simulink model "mpc555_v12_sade_ve_duzenli"  (Simulink 7.0)
settings: Solver=FixedStepDiscrete  StartTime=0.0  StopTime=inf  FixedStep=dt_sys  RelTol=1e-3
PreLoadFcn:
  | RTWConfigurationCB('preloadfcn', bdroot);
InitFcn:
  | % START RTW CONFIGURATION CODE %
  | RTWConfigurationCB('rtw_target_initfcn',gcs);
  | % END RTW CONFIGURATION CODE %
values from neighbouring files (symbols this model uses):
  dt = 1/50    (= 0.02)    [init_par.m]
  dt_serial_RX1 = dt/120    (= 0.000166666666667)    [init_par.m]
  dt_serial_TX2 = dt/120    (= 0.000166666666667)    [init_par.m]
undefined symbols (not defined in the file or in its folder): DiscIntNeverNeededParam
libraries: aerolibconvert2 x9, mpc555drivers x5, simulink x1
(part 2 of 2)

== matlab function Stystem Counter ==
  data: count output inherited
function count  = fcn
% This block supports the Embedded MATLAB subset.
% See the help menu for details. 
persistent counter

if isempty(counter)
    counter =uint16(0);
end

if(counter==65535)
    counter=uint16(0);
end
counter=counter+1;
count=counter;

== matlab function Embedded MATLAB Function ==
  data: a input inherited; P1 output inherited; P2 output inherited; P3 output inherited; b input inherited; c input inherited
function [P1,P2,P3] = fcn(a, b, c)
% This block supports the Embedded MATLAB subset.
% See the help menu for details. 
P1temp = zeros(4,1);
P2temp = zeros(4,1);
P3temp = zeros(4,1);
xP1 = zeros(4,1);
xP2 = zeros(4,1);
xP3 = zeros(4,1);
P1temp(1:4) = typecast(double(a),'int16');
P2temp(1:4) = typecast(double(b),'int16');
P3temp(1:4) = typecast(double(c),'int16');

xP1(1)=P1temp(4);
xP1(2)=P1temp(3);
xP1(3)=P1temp(2);
xP1(4)=P1temp(1);
xP2(1)=P2temp(4);
xP2(2)=P2temp(3);
xP2(3)=P2temp(2);
xP2(4)=P2temp(1);
xP3(1)=P3temp(4);
xP3(2)=P3temp(3);
xP3(3)=P3temp(2);
xP3(4)=P3temp(1);

P1=xP1;
P2=xP2;
P3=xP3;

== matlab function Receive_IMU_Data/Receive Buffer1 ==
  data: Data input uint8; bytes output uint8; endinx output double; Num input double; inbuflen output double
function [bytes, endinx, inbuflen] = buffer(Data, Num)
%inbuflenSC1 length parameter for input buffer
inbuflenSC1 = 170;

persistent rdata inx

% Initialize persistent data
if isempty(rdata)
    rdata = uint8(zeros(inbuflenSC1,1));
end
if isempty(inx)
    inx = 1;
end

% If Data exists
if (Num > 0)
    for inxdata = 1:Num        
        % Grap Data bytes    
        rdata(inx) = Data(inxdata);
        inx = inx + 1;
        if (inx > inbuflenSC1)
            inx = 1;
        end
    end %for
end %if

endinx = inx;
bytes = rdata;
inbuflen = inbuflenSC1;

== matlab function Receive_IMU_Data/IMU B2D ==
  data: dvalid input double; accX output uint16; accY output uint16; accZ output uint16; gyroX output uint16; gyroY output uint16; gyroZ output uint16; magX output uint16; magY output uint16; magZ output uint16; temp output uint16; alt output uint16; airs output uint16; bytes input uint8; temp1 output inherited; temp2 output inherited; temp3 output inherited; temp4 output inherited; temp5 output inherited; temp6 output inherited; temp7 output inherited; temp8 output inherited
function [ accX,accY,accZ,gyroX,gyroY,gyroZ,magX,magY,magZ,temp,alt,airs, temp1, temp2, temp3,temp4, temp5, temp6,temp7, temp8 ] = B2D(dvalid,bytes)

persistent XaccX XaccY XaccZ XgyroX XgyroY XgyroZ XmagX XmagY XmagZ Xtemp Xalt Xairs Xtemp1 Xtemp2 Xtemp3 Xtemp4 Xtemp5 Xtemp6 Xtemp7 Xtemp8 
% Initialize persistent data
if isempty(XaccX)
   XaccX=uint16(0);
end
if isempty(XaccY)
   XaccY=uint16(0);
end
if isempty(XaccZ)
   XaccZ=uint16(0);
end
if isempty(XgyroX)
   XgyroX=uint16(0);
end
if isempty(XgyroY)
   XgyroY=uint16(0);
end
if isempty(XgyroZ)
   XgyroZ=uint16(0);
end
if isempty(XmagX)
   XmagX=uint16(0);
end
if isempty(XmagY)
   XmagY=uint16(0);
end
if isempty(XmagZ)
   XmagZ=uint16(0);
end
if isempty(Xtemp)
   Xtemp=uint16(0);
end
if isempty(Xalt)
   Xalt=uint16(0);
end
if isempty(Xairs)
   Xairs=uint16(0);
end
if isempty(Xtemp1)
   Xtemp1=uint16(0);
end
if isempty(Xtemp2)
   Xtemp2=uint16(0);
end
if isempty(Xtemp3)
   Xtemp3=uint16(0);
end
if isempty(Xtemp4)
   Xtemp4=uint16(0);
end
if isempty(Xtemp5)
   Xtemp5=uint16(0);
end
if isempty(Xtemp6)
   Xtemp6=uint16(0);
end
if isempty(Xtemp7)
   Xtemp7=uint16(0);
end
if isempty(Xtemp8)
   Xtemp8=uint16(0);
end
% accX = zeros(1,1,'uint16');
% accY = zeros(1,1,'uint16');
% accZ = zeros(1,1,'uint16');
% gyroX = zeros(1,1,'uint16');
% gyroY =zeros(1,1,'uint16');
% gyroZ = zeros(1,1,'uint16');
% magX = zeros(1,1,'uint16');
% magY = zeros(1,1,'uint16');
% magZ = zeros(1,1,'uint16');
% temp = zeros(1,1,'uint16');
% alt = zeros(1,1,'uint16');
% airs = zeros(1,1,'uint16');

if (dvalid == 1)
    
  %accX(1)=double(typecast(bytes(2:-1:1),'uint16'));
  
  %accX=[bytes(2); bytes(1)];
    YaccX= typecast(bytes(2:-1:1),'uint16');
    YaccY= typecast(bytes(4:-1:3),'uint16');
    YaccZ= typecast(bytes(6:-1:5),'uint16');
    YgyroX= typecast(bytes(8:-1:7),'uint16');
    YgyroY= typecast(bytes(10:-1:9),'uint16');
    YgyroZ= typecast(bytes(12:-1:11),'uint16');
    YmagX= typecast(bytes(14:-1:13),'uint16');
    YmagY= typecast(bytes(16:-1:15),'uint16');
    YmagZ= typecast(bytes(18:-1:17),'uint16');
    Ytemp= typecast(bytes(20:-1:19),'uint16');
    Yalt= typecast(bytes(22:-1:21),'uint16');
    Yairs= typecast(bytes(24:-1:23),'uint16');
    Ytemp1= typecast(bytes(26:-1:25),'uint16');
    Ytemp2= typecast(bytes(28:-1:27),'uint16');
    Ytemp3= typecast(bytes(30:-1:29),'uint16');
    Ytemp4= typecast(bytes(32:-1:31),'uint16');
    Ytemp5= typecast(bytes(34:-1:33),'uint16');
    Ytemp6= typecast(bytes(36:-1:35),'uint16');
    Ytemp7= typecast(bytes(38:-1:37),'uint16');
    Ytemp8= typecast(bytes(40:-1:39),'uint16');
    
    XaccX=YaccX(1) ;
    XaccY=YaccY(1) ;
    XaccZ=YaccZ(1) ;
    XgyroX=YgyroX(1);
    XgyroY=YgyroY(1);
    XgyroZ=YgyroZ(1);
    XmagX=YmagX(1);
    XmagY=YmagY(1);
    XmagZ=YmagZ(1); 
    Xtemp=Ytemp(1);
    Xalt=Yalt(1);
    Xairs=Yairs(1);
    Xtemp1=Ytemp1(1);
    Xtemp2=Ytemp2(1);
    Xtemp3=Ytemp3(1);
    Xtemp4=Ytemp4(1);
    Xtemp5=Ytemp5(1);
    Xtemp6=Ytemp6(1);
    Xtemp7=Ytemp7(1);
    Xtemp8=Ytemp8(1);
    
    
end
    
    %ivalue = typecast(bytes(24:-1:23),'uint16');
   accX=XaccX ;
   accY=XaccY ;
   accZ=XaccZ ;
   gyroX=XgyroX;
   gyroY=XgyroY;
   gyroZ=XgyroZ;
   magX=XmagX;
   magY=XmagY;
   magZ=XmagZ; 
   temp=Xtemp;
   alt=Xalt;
   airs=Xairs;
   temp1=Xtemp1;
   temp2=Xtemp2;
   temp3=Xtemp3;
   temp4=Xtemp4;
   temp5=Xtemp5;
   temp6=Xtemp6;
    temp7=Xtemp7;
   temp8=Xtemp8;
   % value = uint8(ivalue(1));
%end

== matlab function Receive_IMU_Data/GPS B2D ==
  data: dvalid input inherited; bytes input inherited; Lat_Degrees output inherited; Lat_Mins output uint16; Lat_Fractions output uint16; Lat_Dir output uint16; Lon_Degrees output uint16; Lon_Mins output uint16; Lon_Fractions output uint16; Lon_Dir output uint16; gps_alt output inherited; gps_alt_fraction output inherited; gps_speed output uint16; gps_speed_fraction output uint16; gps_trackangle output uint16; gps_trackangle_fraction output uint16; gps_date output inherited; gps_month output inherited; gps_year output inherited; gps_time_h output double; gps_time_m output inherited; gps_time_s output inherited
function [Lat_Degrees,Lat_Mins,Lat_Fractions,Lat_Dir,Lon_Degrees,Lon_Mins,Lon_Fractions,Lon_Dir,gps_alt, gps_alt_fraction, gps_speed,gps_speed_fraction,gps_trackangle,gps_trackangle_fraction, gps_date, gps_month, gps_year, gps_time_h, gps_time_m, gps_time_s] = B2D(dvalid,bytes)

persistent XLat_Degrees XLat_Mins XLat_Fractions XLat_Dir XLon_Degrees XLon_Mins XLon_Fractions XLon_Dir Xgps_speed Xgps_speed_fraction Xgps_trackangle Xgps_trackangle_fraction Xgps_date Xgps_month Xgps_year Xgps_time_h Xgps_time_m Xgps_time_s Xgps_alt Xgps_alt_fraction

	
% Initialize persistent data
if isempty(XLat_Degrees)
   XLat_Degrees=uint16(0);
end
if isempty(XLat_Mins)
   XLat_Mins=uint16(0);
end
if isempty(XLat_Fractions)
   XLat_Fractions=uint16(0);
end
if isempty(XLat_Dir)
   XLat_Dir=uint16(0);
end
if isempty(XLon_Degrees)
   XLon_Degrees=uint16(0);
end
if isempty(XLon_Mins)
   XLon_Mins=uint16(0);
end
if isempty(XLon_Fractions)
   XLon_Fractions=uint16(0);
end
if isempty(XLon_Dir)
   XLon_Dir=uint16(0);
end
if isempty(Xgps_speed)
   Xgps_speed=uint16(0);
end
if isempty(Xgps_speed_fraction)
   Xgps_speed_fraction=uint16(0);
end
if isempty(Xgps_trackangle)
   Xgps_trackangle=uint16(0);
end
if isempty(Xgps_trackangle_fraction)
   Xgps_trackangle_fraction=uint16(0);
end
if isempty(Xgps_date)
   Xgps_date=uint16(0);
end
if isempty(Xgps_month)
   Xgps_month=uint16(0);
end
if isempty(Xgps_year)
   Xgps_year=uint16(0);
end
if isempty(Xgps_time_h)
   Xgps_time_h=uint16(0);
end
if isempty(Xgps_time_m)
   Xgps_time_m=uint16(0);
end
if isempty(Xgps_time_s)
   Xgps_time_s=uint16(0);
end
if isempty(Xgps_alt)
   Xgps_alt=uint16(0);
end
if isempty(Xgps_alt_fraction)
   Xgps_alt_fraction=uint16(0);
end


% Lat_Degrees = zeros(1,1,'uint16');
% Lat_Mins = zeros(1,1,'uint16');
% Lat_Fractions = zeros(1,1,'uint16');
% Lat_Dir = zeros(1,1,'uint16');
% Lon_Degrees =zeros(1,1,'uint16');
% Lon_Mins = zeros(1,1,'uint16');
% Lon_Fractions = zeros(1,1,'uint16');
% Lon_Dir = zeros(1,1,'uint16');
% gps_speed = zeros(1,1,'uint16');
% gps_speed_fraction = zeros(1,1,'uint16');
% gps_trackangle = zeros(1,1,'uint16');
% gps_trackangle_fraction = zeros(1,1,'uint16');

if (dvalid == 1)
    
  %Lat_Degrees(1)=double(typecast(bytes(2:-1:1),'uint16'));
  
  %Lat_Degrees=[bytes(2); bytes(1)];
    YLat_Degrees= typecast(bytes(2:-1:1),'uint16');
    YLat_Mins= typecast(bytes(4:-1:3),'uint16');
    YLat_Fractions= typecast(bytes(6:-1:5),'uint16');
    YLat_Dir= typecast(bytes(8:-1:7),'uint16');
    YLon_Degrees= typecast(bytes(10:-1:9),'uint16');
    YLon_Mins= typecast(bytes(12:-1:11),'uint16');
    YLon_Fractions= typecast(bytes(14:-1:13),'uint16');
    YLon_Dir= typecast(bytes(16:-1:15),'uint16');
    Ygps_alt= typecast(bytes(18:-1:17),'uint16');
    Ygps_alt_fraction= typecast(bytes(20:-1:19),'uint16');
    Ygps_speed= typecast(bytes(22:-1:21),'uint16');
    Ygps_speed_fraction= typecast(bytes(24:-1:23),'uint16');
    Ygps_trackangle= typecast(bytes(26:-1:25),'uint16');
    Ygps_trackangle_fraction= typecast(bytes(28:-1:27),'uint16');
    Ygps_date= typecast(bytes(30:-1:29),'uint16');
    Ygps_month= typecast(bytes(32:-1:31),'uint16');
    Ygps_year= typecast(bytes(34:-1:33),'uint16');
    Ygps_time_h= typecast(bytes(36:-1:35),'uint16');
    Ygps_time_m= typecast(bytes(38:-1:37),'uint16');
    Ygps_time_s= typecast(bytes(40:-1:39),'uint16');
    
    
    
    XLat_Degrees=YLat_Degrees(1) ;
    XLat_Mins=YLat_Mins(1) ;
    XLat_Fractions=YLat_Fractions(1) ;
    XLat_Dir=YLat_Dir(1);
    XLon_Degrees=YLon_Degrees(1);
    XLon_Mins=YLon_Mins(1);
    XLon_Fractions=YLon_Fractions(1);
    XLon_Dir=YLon_Dir(1);
    Xgps_speed=Ygps_speed(1); 
    Xgps_speed_fraction=Ygps_speed_fraction(1);
    Xgps_trackangle=Ygps_trackangle(1);
    Xgps_trackangle_fraction=Ygps_trackangle_fraction(1);
    Xgps_date=Ygps_date(1);
    Xgps_month=Ygps_month(1);
    Xgps_year=Ygps_year(1);
    Xgps_time_h=Ygps_time_h(1);
    Xgps_time_m=Ygps_time_m(1);
    Xgps_time_s=Ygps_time_s(1);
    Xgps_alt=Ygps_alt(1);
    Xgps_alt_fraction=Ygps_alt_fraction(1);
    
    
end
    
    %ivalue = typecast(bytes(24:-1:23),'uint16');
   Lat_Degrees=XLat_Degrees ;
   Lat_Mins=XLat_Mins ;
   Lat_Fractions=XLat_Fractions ;
   Lat_Dir=XLat_Dir;
   Lon_Degrees=XLon_Degrees;
   Lon_Mins=XLon_Mins;
   Lon_Fractions=XLon_Fractions;
   Lon_Dir=XLon_Dir;
   gps_speed=Xgps_speed; 
   gps_speed_fraction=Xgps_speed_fraction;
   gps_trackangle=Xgps_trackangle;
   gps_trackangle_fraction=Xgps_trackangle_fraction;
   gps_date=Xgps_date;
   gps_month=Xgps_month;
   gps_year=Xgps_year;
   gps_time_h=Xgps_time_h;
   gps_time_m=Xgps_time_m;
   gps_time_s=Xgps_time_s;
   gps_alt=Xgps_alt;
   gps_alt_fraction=Xgps_alt_fraction;
   % value = uint8(ivalue(1));
%end

== matlab function Receive_IMU_Data/Read Buffer2 ==
  data: dvalid output double; imu_data output double; bytes input uint8; endinx input double; inbuflenSC2 input double
function [dvalid, imu_data] = fcn(bytes, endinx, inbuflenSC2)
%inbuflenSC2 length parameter for input buffer

persistent indata inx curinx 


%Constants 
headerlen = 2;
dlen = 40;
cslen = 2;

% Initialize persistent data
if isempty(indata)
    indata = zeros(dlen,1,'uint8');
end
if isempty(inx)
    inx = 1;
end
if isempty(curinx)
    curinx = 1;
end

outbuf = uint8(zeros(dlen,1));

dvalid = uint8(0);
%
while ((endinx ~= 0) && (inx ~= endinx))
    if (curinx == 1)
        if (bytes(inx) == 255) %0xFF
            curinx = curinx + 1;
        else
            curinx=1;
        end       
    elseif (curinx == 2)
        if (bytes(inx) == 251) %0xFB
            curinx = curinx + 1;
        elseif (bytes(inx) == 255) %0xFF
            curinx = 2;
        else
            curinx = 1;
        end
    elseif (curinx == 43)
        if (bytes(inx) == 13) %0x0D
            curinx = curinx + 1;
        else
            curinx = 1;
        end
    elseif (curinx == 44)   % Last data received       
        if (bytes(inx) == 10) %0x0A
            outbuf = indata;    % Copy received data to output buffer            
        %    dvalid = dvalid + uint8(1);         % This data is valid and fresh
            dvalid =uint8(1);         % This data is valid and fresh
        end              
        curinx = 1; % Reset counter             
    else    % Grap Data bytes  
        indata(curinx-headerlen) = bytes(inx);
        curinx = curinx + 1;
    end       
    
    inx = inx + 1;
    if (inx > inbuflenSC2)
        inx = 1;
    end
end

imu_data = outbuf(1:dlen);

== matlab function Butunlesik Seyir Sistemi/Hesaplamalar/INS/GPS Hiz Bilesenleri ==
  data: gpsspeed input double; Vx output double; gpsheading input double; Vy output double
function [Vx,Vy] = fcn(gpsspeed,gpsheading)
%#eml

 Vx=gpsspeed*cos(gpsheading*(3.14159/180.00));
  Vy=gpsspeed*sin(gpsheading*(3.14159/180.00));

== matlab function Butunlesik Seyir Sistemi/Hesaplamalar/INS/Govde-Seyrusefer Eksen Donusumu ==
  data: accx input double; accy input double; accz input double; roll input double; aN output double; pitch input double; yaw input double; aE output double; aD output double
function [aN,aE,aD] = fcn(accx,accy,accz,roll,pitch,yaw)
%#eml

persistent Macc  sample_counter ax ay az aN_correction aE_correction aD_correction cal_finished Y;

num_of_sample=100;

% Initialize persistent data
if isempty(Macc)
    Macc = [0;0;0];
end

if isempty(sample_counter)
    sample_counter = 0;
end

if isempty(ax)
    ax = 0;
end

if isempty(ay)
    ay = 0;
end

if isempty(az)
    az = 0;
end

if isempty(aN_correction)
    aN_correction = 0;
end
if isempty(aE_correction)
    aE_correction = 0;
end
if isempty(aD_correction)
    aD_correction = 0;
end
if isempty(cal_finished)
    cal_finished = 0;
end
if isempty(Y)
    Y =[0;0;0];
end

if(sample_counter<num_of_sample)
   if(sample_counter>10)
   ax=ax+accx;
   ay=ay+accy;
   az=az+accz;
   end
   sample_counter=sample_counter+1;
end

%%%%%%%%%%%%%%%%%%%Calibration Routine%%%%%%%%%%%%%%%%%%%%%%
if(sample_counter==num_of_sample)
    aN_correction=ax/(num_of_sample-11);
    aE_correction=ay/(num_of_sample-11);
    aD_correction=az/(num_of_sample-11);
    cal_finished=1;
    sample_counter=sample_counter+1;
end
%%%%%%%%%%%%%%%%%%%%%%%%%%%%%%%%%%%%%%%%%%%%%%%%%%%%%%%%%%%%%

if(cal_finished==1)
Macc(1,1)=accx;
Macc(2,1)=-accy;
Macc(3,1)=accz;

%DCM matris Body to Navigation Frame
M2=[ cos(pitch)*cos(yaw)   (sin(roll)*sin(pitch)*cos(yaw)- cos(roll)*sin(yaw))    (cos(roll)*sin(pitch)*cos(yaw)+ sin(roll)*sin(yaw)) ;
    cos(pitch)*sin(yaw)    (sin(roll)*sin(pitch)*sin(yaw)+ cos(roll)*cos(yaw))    (cos(roll)*sin(pitch)*sin(yaw)- sin(roll)*cos(yaw));
    -sin(pitch)                         (sin(roll)*cos(pitch))                                (cos(roll)*cos(pitch))];

% M2=[ 1   tan(pitch)*sin(roll)    tan(pitch)*cos(roll)  ;
%     0       cos(roll)                -sin(roll)       ;
%     0   (sin(roll)/cos(pitch))  (cos(roll)/cos(pitch))];

Y=M2*Macc;
end
aN=Y(1,1)-aN_correction;
aE=Y(2,1)-aE_correction;
aD=-((Y(3,1))-aD_correction);

== matlab function Butunlesik Seyir Sistemi/Gercek Birimleri Hesapla/Manyetometre ==
  data: RAWmagX input double; magX output double; RAWmagY input double; RAWmagZ input double; magY output double; magZ output double; X_MIN output double; X_MAX output double; Y_MIN output double; Y_MAX output double; Z_MIN output double; Z_MAX output double; XScale output double; YScale output double; Xoff output double; Yoff output double; CAL_EN input double

function [magX,magY,magZ,X_MIN, X_MAX, Y_MIN, Y_MAX, Z_MIN, Z_MAX, XScale,YScale, Xoff,Yoff ] = fcn(RAWmagX,RAWmagY,RAWmagZ, CAL_EN )
%#eml


persistent RmagX_MIN RmagX_MAX RmagY_MIN RmagY_MAX RmagZ_MIN RmagZ_MAX XRange YRange ZRange Xsf Ysf Zsf X_off Y_off Z_off Xold Yold Zold RAWmX RAWmY RAWmZ first_time cal_done count
%persistent Xtemp Ytemp Ztemp
%persistent roll pitch

% Initialize persistent data
if isempty(RmagX_MIN)
    RmagX_MIN = double(4095);
end

if isempty(RmagX_MAX)
    RmagX_MAX = double(0);
end

if isempty(RmagY_MIN)
    RmagY_MIN = double(4095);
end

if isempty(RmagY_MAX)
    RmagY_MAX =double(0);
end

if isempty(RmagZ_MIN)
    RmagZ_MIN = double(4095);
end

if isempty(RmagZ_MAX)
    RmagZ_MAX = double(0);
end

if isempty(Xsf)
    Xsf = double(1);
end
if isempty(Ysf)
    Ysf = double(1);
end
if isempty(Zsf)
    Zsf = double(1);
end
if isempty(X_off)
    X_off = double(136);
end
if isempty(Y_off)
    Y_off = double(136);
end
if isempty(Z_off)
    Z_off = double(136);
end

if isempty(Xold)
    Xold = RAWmagX;
end
if isempty(Yold)
    Yold = RAWmagY;
end
if isempty(Zold)
    Zold = RAWmagZ;
end

if isempty(RAWmX)
    RAWmX = RAWmagX;
end

if isempty(RAWmY)
    RAWmY = RAWmagY;
end

if isempty(RAWmZ)
    RAWmZ = RAWmagZ;
end

if isempty(XRange)
    XRange =double(192);
end

if isempty(YRange)
    YRange =double(160);
end

if isempty(ZRange)
    ZRange =double(192);
end

if isempty(first_time)
    first_time = double(1);
end

if isempty(cal_done)
    cal_done = double(0);
end

if isempty(count)
    count = uint16(0);
end
%%%%%%%%%%%%%%Filter the data%%%%%%%%%%%%%%%%
if(count<100)
    count=count+1;
end
    
   if(count>=100)
       if(abs(RAWmagX-Xold)< 50)
            RAWmX=RAWmagX;
            Xold=RAWmX;
        else
            RAWmX=Xold;
        end

        if(abs(RAWmagY-Yold)< 50)
            RAWmY=RAWmagY;
            Yold=RAWmY;
        else
            RAWmY=Yold;
        end

        if(abs(RAWmagZ-Zold)< 50)
            RAWmZ=RAWmagZ;
            Zold=RAWmZ;
        else
            RAWmZ=Zold;
        end
   
   else
    RAWmX=RAWmagX;
    Xold=RAWmX;
    RAWmY=RAWmagY;
    Yold=RAWmY;
    RAWmZ=RAWmagZ;
    Zold=RAWmZ;   
   end

    if(CAL_EN==1)
        if(RAWmX>RmagX_MAX)
            RmagX_MAX=RAWmX;
        end
        if(RAWmX<RmagX_MIN)
            RmagX_MIN=RAWmX;
        end
        if(RAWmY>RmagY_MAX)
            RmagY_MAX=RAWmY;
        end
        if(RAWmY<RmagY_MIN)
            RmagY_MIN=RAWmY;
        end
        if(RAWmZ>RmagZ_MAX)
            RmagZ_MAX=RAWmZ;
        end
        if(RAWmZ<RmagZ_MIN)
            RmagZ_MIN=RAWmZ;
        end

        XRange= RmagX_MAX-RmagX_MIN;
        YRange= RmagY_MAX-RmagY_MIN;
        ZRange= RmagZ_MAX-RmagZ_MIN;

        
        magX=double(0);
        magY=double(0);
        magZ=double(0);

        XScale=double(0);
        YScale=double(0);

        Xoff=double(0);
        Yoff=double(0);

        X_MIN=RmagX_MIN;
        X_MAX=RmagX_MAX;
        Y_MIN=RmagY_MIN;
        Y_MAX=RmagY_MAX;
        Z_MIN=RmagZ_MIN;
        Z_MAX=RmagZ_MAX;
        
       cal_done=1;

    else
      %  if(CAL_EN==0)
%     Xtemp= RAWmagX-(1794+(290/2.00));
%     Ytemp= RAWmagY-(2325+(250/2.00));
%     Ztemp= RAWmagZ-(1984+(300/2.00));
    
        if(first_time==1 && cal_done==1)
           if(Xsf< (YRange/XRange))
                Xsf=(YRange/XRange);
            end
            if(Ysf< (XRange/YRange))
                Ysf=(XRange/YRange);
            end

%             X_off= (XRange/2.00 + RmagX_MIN)*Xsf;
%             Y_off= (YRange/2.00 + RmagY_MIN)*Ysf;
%             Z_off= (ZRange/2.00 + RmagZ_MIN)*Zsf;
%             
            X_off= (XRange/2.00)*Xsf;
            Y_off= (YRange/2.00)*Ysf;
            Z_off= (ZRange/2.00)*Zsf;

            first_time=0;
           % cal_done=0;
        end
        
        
      if(cal_done==0)
%          Xsf=double(1); 
%          Ysf=double(1.411);
%          Zsf=double(1);
%          X_off=100;
%          Y_off=100;  %97.5  <sekilller Xoff=160 Yoff=150 ye gore cizildi
%          Z_off=91.5;
%          RmagX_MIN=1878;  %1878
%          RmagY_MIN=2360;  %2360
%          RmagZ_MIN=2005;
%          RmagX_MAX=2073;  %2073
%          RmagY_MAX=2521;  %2521
%          RmagZ_MAX=2080;   %   
         
         
         Xsf=double(1.11); 
         Ysf=double(1.411);
         Zsf=double(1);
         X_off=250;
         Y_off=450;  %97.5  <sekilller Xoff=160 Yoff=150 ye gore cizildi
         Z_off=350;
         RmagX_MIN=1848;  %1878
         RmagY_MIN=2213;  %2360
         RmagZ_MIN=1979;
         RmagX_MAX=2118;  %2073
         RmagY_MAX=2521;  %2521
         RmagZ_MAX=2295;   % 
         
         
      end
      Xtemp=Xsf*(RAWmX-(RmagX_MIN+(X_off/2)));
      Ytemp=Ysf*(RAWmY-(RmagY_MIN+(Y_off/2))) ;
      Ztemp=Zsf*(RAWmZ-(RmagZ_MIN+(Z_off/2))) ;   



        
%     Xtemp= RAWmX-(1834+((2100-1834)/2.00));
%     Ytemp= RAWmY-(2239+((2480-2239)/2.00));
%     Ztemp= RAWmZ-(1792+((2073-1792)/2.00));
    
        magX=Xtemp;
        magY=Ytemp;
        magZ=-1.1*Ztemp+10;

        XScale=Xsf;
        YScale=Ysf;

        Xoff=X_off;
        Yoff=Y_off;

        X_MIN=RmagX_MIN;
        X_MAX=RmagX_MAX;
        Y_MIN=RmagY_MIN;
        Y_MAX=RmagY_MAX;
        Z_MIN=RmagZ_MIN;
        Z_MAX=RmagZ_MAX;

    
    end

== matlab function Butunlesik Seyir Sistemi/Gercek Birimleri Hesapla/GPS ==
  data: LatDeg input double; Lat output double; LatMin input double; LatFrac input double; Lon output double; LonDeg input double; LonMin input double; LonFrac input double; Alt input double; GPSalt output double; Alt_frac input double; speed input double; speed_frac input double; GPSSpeed output double; trackangle input double; trackangle_frac input double; GPSHeading output double
function [Lat,Lon, GPSalt, GPSSpeed, GPSHeading] = fcn(LatDeg,LatMin,LatFrac,LonDeg,LonMin,LonFrac,Alt, Alt_frac, speed, speed_frac, trackangle,trackangle_frac)
%#eml

%Convert Degrees Minutes to Decimal Degreees
Lat=double(LatDeg)+ (double(LatMin)+ double(LatFrac)/10000.00)/60.00;
Lon=double(LonDeg)+ (double(LonMin)+ double(LonFrac)/10000.00)/60.00;
GPSalt=double(Alt);
GPSSpeed=double(speed);
GPSHeading=double(trackangle);

== matlab function Butunlesik Seyir Sistemi/Gercek Birimleri Hesapla/ivme/Kalibrasyon ==
  data: RAWaccx input double; RAWaccy input double; RAWaccz input double; accx output double; accy output double; accz output double; BIASaccx output double; BIASaccy output double; BIASaccz output double; cal_en input double
function [accx,accy,accz,BIASaccx,BIASaccy,BIASaccz] = fcn(RAWaccx,RAWaccy,RAWaccz, cal_en)
%#eml

persistent sample_counter Baccx Baccy Baccz Baccxtemp Baccytemp Baccztemp cal_finished;

num_of_sample=100;

% Initialize persistent data
if isempty(sample_counter)
    sample_counter = 0;
end

if isempty(Baccx)
    %Baccx = 1980;
    %Baccx = 1975;
    Baccx = 1985;
end

if isempty(Baccy)
    %Baccy = 2273;
    %Baccy = 2280;
    Baccy = 2240;
end

if isempty(Baccz)
    %Baccz = 2310;
    %Baccz = 2040;
    Baccz = 2050;
end

if isempty(cal_finished)
    cal_finished = 0;
end

if isempty(Baccxtemp)
    Baccxtemp = 1980;
end

if isempty(Baccytemp)
    Baccytemp = 2273;
end

if isempty(Baccztemp)
    Baccztemp = 2310;
end


if(cal_en==1)
    if(sample_counter<num_of_sample)
       Baccxtemp=Baccxtemp+double(RAWaccx);
       Baccytemp=Baccytemp+double(RAWaccy);
       Baccztemp=Baccztemp+double(RAWaccz);
       sample_counter=sample_counter+1;
    end

    %%%%%%%%%%%%%%%%%%%Calibration Routine%%%%%%%%%%%%%%%%%%%%%%
    if(sample_counter==num_of_sample)
        Baccx=Baccxtemp/num_of_sample;
        Baccy=Baccytemp/num_of_sample;
        Baccz=(Baccztemp/num_of_sample)-744.546;
        cal_finished=1;
        sample_counter=sample_counter+1;
    end
    
    accx=0;
    accy=0;
    accz=1;
end

    
%%%%%%%%%%%%%%%%%%%%%%%%%%%%%%%%%%%%%%%%%%%%%%%%%%%%%%%%%%%%%
BIASaccx=Baccx;
BIASaccy=Baccy;
BIASaccz=Baccz;
accx=double(RAWaccx)-BIASaccx;
accy=double(RAWaccy)-BIASaccy;
accz=double(RAWaccz)-BIASaccz;

== matlab function Butunlesik Seyir Sistemi/Hesaplamalar/Air Data Computer ==
  data: AirData input double; BaroAltitude output double; TAS output double; IAS output double; Baroset input double; Temperature output double
function [BaroAltitude,TAS,IAS,Temperature] = fcn(AirData, Baroset)
%#eml

BIASalt=200.00; %m
BIASairs=185.00; %mV;
bit_weight=0.80586;


static_res_divider=1.99558;
dynamic_res_divider=2.0408;
pressure_sea_level=101.325; %kPa

air_gas_constant=8.31432;
air_density_sea_level=1.225;
absolute_null_kelvin=273.15;

static_press_in_kpa=AirData(2)-Baroset;
diff_press_in_kpa= AirData(3);
temp_celcius=  AirData(1);   

%alt=44330.0 * ((1-((static_press_in_kpa/pressure_sea_level)^(1/5.255))));



IAS_in_m_s=sqrt((2.0*abs(diff_press_in_kpa))/air_density_sea_level); % m/sn
IAS_in_km_h=3.6*IAS_in_m_s;

air_density= static_press_in_kpa/(air_gas_constant * (temp_celcius + absolute_null_kelvin));

TAS_in_m_s= IAS_in_m_s * sqrt(air_density_sea_level/air_density);
TAS_in_km_h= TAS_in_m_s * 3.6;

altitude_in_feet= (1-((static_press_in_kpa*10)/1013.25)^0.190284)*145366.45;
altitude_in_m=0.3048*altitude_in_feet;


BaroAltitude=altitude_in_m;
Temperature=temp_celcius;
IAS=IAS_in_km_h;
TAS=TAS_in_km_h-8; % 8 for calibration

== matlab function Butunlesik Seyir Sistemi/Hesaplamalar/Yonelim ve Bas Acisi Hesaplama/Attitude Computer2/Embedded MATLAB Function2 ==
  data: ay output double; accY input double; accZ input double; roll input double
function ay  = f(accY,accZ,roll)
%#eml

if(accY>0 && accZ>0 && roll>1.0)
    ay=9.8+accZ;
elseif(accY<0 && accZ>0 && roll<-1.0)
    ay=-9.8+-accZ;
    else
        ay=accY;
end
  
% 
% if(roll>1.569)
%     ay=9.8+accZ;
% elseif(roll<-1.569)
%     ay=-9.8+-accZ;
%     else
%         ay=accY;
% end

== matlab function Receive_IMU_Data/Read Buffer1 ==
  data: dvalid output double; imu_data output double; bytes input uint8; endinx input double; inbuflenSC2 input double
function [dvalid, imu_data] = fcn(bytes, endinx, inbuflenSC2)
%inbuflenSC2 length parameter for input buffer

persistent indata inx curinx 


%Constants 
headerlen = 2;
dlen = 40;
cslen = 2;

% Initialize persistent data
if isempty(indata)
    indata = zeros(dlen,1,'uint8');
end
if isempty(inx)
    inx = 1;
end
if isempty(curinx)
    curinx = 1;
end

outbuf = uint8(zeros(dlen,1));

dvalid = uint8(0);
%
while ((endinx ~= 0) && (inx ~= endinx))
    if (curinx == 1)
        if (bytes(inx) == 255) %0xFF
            curinx = curinx + 1;
        else
            curinx=1;
        end       
    elseif (curinx == 2)
        if (bytes(inx) == 250) %0xFA
            curinx = curinx + 1;
        elseif (bytes(inx) == 255) %0xFF
            curinx = 2;
        else
            curinx = 1;
        end
    elseif (curinx == 43)
        if (bytes(inx) == 13) %0x0D
            curinx = curinx + 1;
        else
            curinx = 1;
        end
    elseif (curinx == 44)   % Last data received       
        if (bytes(inx) == 10) %0x0A
            outbuf = indata;    % Copy received data to output buffer            
        %    dvalid = dvalid + uint8(1);         % This data is valid and fresh
            dvalid =uint8(1);         % This data is valid and fresh
        end              
        curinx = 1; % Reset counter             
    else    % Grap Data bytes  
        indata(curinx-headerlen) = bytes(inx);
        curinx = curinx + 1;
    end       
    
    inx = inx + 1;
    if (inx > inbuflenSC2)
        inx = 1;
    end
end

imu_data = outbuf(1:dlen);

== matlab function Send_AHRS_Data/Transmit2/Serialize ==
  data: bytes input double; sync input double; Data output double; Req output double
function [Data, Req]  = fun(bytes, sync)

persistent inx syncsig

if isempty(inx)
    inx = length(bytes) + 1;
end
if isempty(syncsig)
    syncsig = uint8(0);
end
 
Data = uint8(0);
Req = uint32(0);

if (syncsig ~= sync)
    syncsig = sync;
    inx = 1;
end

if (inx <= length(bytes))
    Req = uint32(1);
    Data = bytes(inx);
    inx = inx + 1;
end

== matlab function Butunlesik Seyir Sistemi/Hesaplamalar/Yonelim ve Bas Acisi Hesaplama/Kuzey Acisi Hesaplama ==
  data: x output double; y output double; z output double; mag input double; attitude input double size=3; Declination input double; Xh output double; Yh output double; MagneticHeading output double; TrueHeading output double size=1; x1 output double; x2 output double; x3 output double; y1 output double; y2 output double
function [x,y,z, Xh, Yh, MagneticHeading,TrueHeading,x1,x2,x3,y1,y2] = fcn(mag,attitude,Declination)
%#eml

mX=mag(1)+5;
%mY=mag(2)+150;
mY=mag(2);
mZ=mag(3);
x=mX;
y=mY;
z=mZ;
roll=(attitude(1)*0.01745); %in rad
pitch=(attitude(2)*0.01745); % in rad

% x1=mX*cos(pitch);
% x2=mY*1.2*sin(roll)*sin(pitch);
% x3=- mZ*cos(roll)*sin(pitch);
% 
% y1= mY*1.2*cos(roll);
% y2=mZ*sin(roll);
% 
% Xh=x1+x2+x3;
% Yh=y1+y2;
% 

x1=0;
x2=0;
x3=0;
y1=0;
y2=0;
Xh = mX*cos(pitch) + mY*sin(roll)*sin(pitch) + mZ*cos(roll)*sin(pitch);
Yh = mY*cos(roll) - mZ*sin(roll);

% Xh = mX*cos(pitch) + mY*sin(roll)*sin(pitch) + mZ*cos(pitch)*sin(roll);
% Yh = mY*cos(pitch) - mZ*sin(pitch);


%MagneticHeading = ((atan2(-mY,mX))*57.2957);
MagneticHeading = ((atan2(-Yh,Xh))*57.2957);
TrueHeading = MagneticHeading+ Declination;

== matlab function Send_AHRS_Data/Put in array ==
  data: dvalid input double; bytes input double; bytes1 output double; sync output double
function [bytes1, sync] = fcn(dvalid, bytes)

persistent syncsig count sbytes bytesbuffer

% Initialize persistent data
if isempty(syncsig)
    syncsig = uint8(0);
end
if isempty(count)
    count = uint8(0);
end
if isempty(sbytes)
    sbytes = uint8(zeros(104,1));
end

% if isempty(bytesbuffer)
%     bytesbuffer = uint8(zeros(70,1));
% end


%if (dvalid == 1)    
%if (dvalid == 1 )
    %bytesbuffer=typecast(bytes,'uint8');
     accX= typecast(bytes(1),'uint8');
     accY= typecast(bytes(2),'uint8');
     accZ= typecast(bytes(3),'uint8');
     gyroX= typecast(bytes(4),'uint8');
     gyroY= typecast(bytes(5),'uint8');
     gyroZ= typecast(bytes(6),'uint8');
     magX= typecast(bytes(7),'uint8');
     magY= typecast(bytes(8),'uint8');
     magZ= typecast(bytes(9),'uint8');
     temp= typecast(bytes(10),'uint8');
     alt= typecast(bytes(11),'uint8');
     ias= typecast(bytes(12),'uint8');
     roll= typecast(bytes(13),'uint8');
     pitch= typecast(bytes(14),'uint8');
     yaw= typecast(bytes(15),'uint8');  
     temp1=typecast(bytes(16),'uint8');
     temp2=typecast(bytes(17),'uint8');
     temp3=typecast(bytes(18),'uint8');
     temp4=typecast(bytes(19),'uint8');
     temp5=typecast(bytes(20),'uint8');
     Lat_Degrees=typecast(bytes(21),'uint8');
     Lat_Mins=typecast(bytes(22),'uint8');
     Lat_Fractions=typecast(bytes(23),'uint8');
     Lat_Dir=typecast(bytes(24),'uint8');
     Lon_Degrees=typecast(bytes(25),'uint8');
     Lon_Mins=typecast(bytes(26),'uint8');
     Lon_Fractions=typecast(bytes(27),'uint8');
     Lon_Dir=typecast(bytes(28),'uint8');
     gps_speed=typecast(bytes(29),'uint8');
     gps_speed_fraction=typecast(bytes(30),'uint8');
     gps_trackangle=typecast(bytes(31),'uint8');
     gps_trackangle_fraction=typecast(bytes(32),'uint8');
     gps_date=typecast(bytes(33),'uint8');
     gps_month=typecast(bytes(34),'uint8');
     gps_year=typecast(bytes(35),'uint8');
     gps_time_h=typecast(bytes(36),'uint8');
     gps_time_m=typecast(bytes(37),'uint8');
     gps_time_s=typecast(bytes(38),'uint8');
     gps_alt=typecast(bytes(39),'uint8');
     gps_alt_fraction=typecast(bytes(40),'uint8');
     d41=typecast(bytes(41),'uint8');
     d42=typecast(bytes(42),'uint8');
     d43=typecast(bytes(43),'uint8');
     d44=typecast(bytes(44),'uint8');
     d45=typecast(bytes(45),'uint8');
     d46=typecast(bytes(46),'uint8');
     d47=typecast(bytes(47),'uint8');
     d48=typecast(bytes(48),'uint8');
     d49=typecast(bytes(49),'uint8');
     d50=typecast(bytes(50),'uint8');
         
    sbytes(1:104) = [255; 250; 
                    accX(2); accX(1); accY(2); accY(1);accZ(2); accZ(1); 
                    gyroX(2); gyroX(1);gyroY(2); gyroY(1);gyroZ(2); gyroZ(1);
                    magX(2); magX(1);magY(2); magY(1); magZ(2); magZ(1);
                    temp(2); temp(1);alt(2); alt(1);ias(2); ias(1);
                    roll(2); roll(1);pitch(2); pitch(1);yaw(2); yaw(1);
                    temp1(2);temp1(1);temp2(2);temp2(1);temp3(2);temp3(1);temp4(2);temp4(1);temp5(2);temp5(1);
                    Lat_Degrees(2);Lat_Degrees(1);Lat_Mins(2);Lat_Mins(1);
                    Lat_Fractions(2);Lat_Fractions(1);Lat_Dir(2);Lat_Dir(1);
                    Lon_Degrees(2);Lon_Degrees(1);Lon_Mins(2);Lon_Mins(1);
                    Lon_Fractions(2);Lon_Fractions(1);Lon_Dir(2);Lon_Dir(1);
                    gps_speed(2);gps_speed(1);gps_speed_fraction(2);gps_speed_fraction(1);
                    gps_trackangle(2);gps_trackangle(1);gps_trackangle_fraction(2);gps_trackangle_fraction(1);
                    gps_date(2);gps_date(1);gps_month(2);gps_month(1);gps_year(2);gps_year(1);
                    gps_time_h(2);gps_time_h(1); gps_time_m(2);gps_time_m(1); gps_time_s(2);gps_time_s(1);
                    gps_alt(2);gps_alt(1);gps_alt_fraction(2);gps_alt_fraction(1);
                    d41(2);d41(1); d42(2);d42(1); d43(2);d43(1); d44(2);d44(1); d45(2);d45(1); d46(2);d46(1);
                    d47(2);d47(1); d48(2);d48(1); d49(2);d49(1); d50(2);d50(1);
                    13; 10];
%else
   % sbytes = [255; 250; uint8(zeros(24,1))];    

%end

if (syncsig == 0)
    syncsig = uint8(1);
else
    syncsig = uint8(0);
end


% if (count == 0)
%     count = uint8(1);
% %elseif (count == 1)
% %    count = uint8(2);
% else
%     count = uint8(0);
% end

bytes1 = sbytes;
sync = syncsig;

== matlab function Butunlesik Seyir Sistemi/Hesaplamalar/Yonelim ve Bas Acisi Hesaplama/Attitude Computer2/DCM ==
  data: p input double size=1; q input double size=1; r input double size=1; roll input double size=1; roll_rate output double size=1; pitch input double size=1; yaw input double size=1; pitch_rate output double size=1; yaw_rate output double size=1
function [roll_rate,pitch_rate,yaw_rate] = fcn(p,q,r,roll,pitch,yaw)
%Durum(Oryantasyon Hesaplama

Mgyro=[0;0;0];
Mgyro(1,1)=p;
Mgyro(2,1)=q;
Mgyro(3,1)=r;

% M=[ 1   tan(pitch)*sin(roll)    tan(pitch)*cos(roll)  ;
%     0       cos(roll)                -sin(roll)       ;
%     0   (sin(roll)/cos(pitch))  (cos(roll)/cos(pitch))];

M=[ 1   tan(pitch)*sin(roll)    tan(pitch)*cos(roll)  ;
    0       cos(roll)                -sin(roll)       ;
    0   (sin(roll)/sec(pitch))  (cos(roll)/sec(pitch))];

m11=M(1,1);
m12=M(1,2);
m13=M(1,3);

Y=M*Mgyro;     

roll_rate=Y(1,1);
pitch_rate=Y(2,1);
yaw_rate=Y(3,1);

== matlab function Butunlesik Seyir Sistemi/Hesaplamalar/Yonelim ve Bas Acisi Hesaplama/Attitude Computer2/Embedded MATLAB Function1 ==
  data: ayc output double; roll input double; axc output double; pitch input double; yaw input double; azc output double
function [ayc,axc,azc] = fcn(roll,pitch,yaw)
%#eml
g=9.8;
axc=g*sin(pitch);
%ayc=g*cos(roll-pi/2);  % My correction
% if(roll>1.553)
%         ayc=g*(1+sin(roll-1.57));  % My correction
% elseif(roll<-1.553)
%         ayc=g*(-1+sin(roll+1.57));  % My correction
% else
%     ayc=g*sin(roll);  % My correction
% end

if(roll>1.569)
        ayc=g+g*(sin(roll-1.569));  % My correction
elseif(roll<-1.569)
        ayc=-g+g*(sin(roll+1.569));  % My correction
else
    ayc=g*sin(roll);  % My correction
end

%ayc=-g*(cos(pitch)*sin(roll)); %Notes
%azc=-g*cos(pitch)*cos(roll);
azc=yaw;

== matlab function Butunlesik Seyir Sistemi/Hesaplamalar/Yonelim ve Bas Acisi Hesaplama/filter ==
  data: u input double; y output double
function y = f(u)
%#eml

persistent u1 u2 u3 u4 u5 u6 u7 u8 u9 u10

if isempty(u1)
    u1 = [double(0);double(0);double(0)];
    u2 = [double(0);double(0);double(0)];
    u3 = [double(0);double(0);double(0)];
    u4 = [double(0);double(0);double(0)];
    u5 = [double(0);double(0);double(0)];
    u6 = [double(0);double(0);double(0)];
    u7 = [double(0);double(0);double(0)];
    u8 = [double(0);double(0);double(0)];
    u9 = [double(0);double(0);double(0)];
    u10 = [double(0);double(0);double(0)];
end
u10=u9;
u9=u8;
u8=u7;
u7=u6;
u6=u5;
u5=u4;
u4=u3;
u3=u2;
u2=u1;
u1=u;

y =(u1+u2+u3+u4+u5+u6+u7+u8+u9+u10)/10.0;

== matlab function Butunlesik Seyir Sistemi/Hesaplamalar/INS/INS Vertical Channel/Embedded MATLAB Function1 ==
  data: u input double; y output double
function y = g(u)
%#eml

go=9.78; %m/s^2
Ro=6378000; %m

y =((2*go)/Ro)* u;

== matlab function Butunlesik Seyir Sistemi/Hesaplamalar/Yonelim ve Bas Acisi Hesaplama/filter7 ==
  data: u input double; y output double
function y = f(u)
%#eml

persistent u1 u2 u3 u4 u5 u6 u7 u8 u9 u10

if isempty(u1)
    u1 = double(0);
    u2 = double(0);
    u3 = double(0);
    u4 = double(0);
    u5 = double(0);
    u6 = double(0);
    u7 = double(0);
    u8 = double(0);
    u9 = double(0);
    u10 = double(0);
end

u10=u9;
u9=u8;
u8=u7;
u7=u6;
u6=u5;
u5=u4;
u4=u3;
u3=u2;
u2=u1;
u1=u;

y =(u1+u2+u3+u4+u5+u6+u7+u8+u9+u10)/10.0;

== matlab function Butunlesik Seyir Sistemi/Hesaplamalar/filter2 ==
  data: u input double; y output double
function y = f(u)
%#eml

persistent u1 u2 u3 u4 u5 u6 u7 u8 u9 u10

if isempty(u1)
    u1 = double(0);
    u2 = double(0);
    u3 = double(0);
    u4 = double(0);
    u5 = double(0);
    u6 = double(0);
    u7 = double(0);
    u8 = double(0);
    u9 = double(0);
    u10 = double(0);
end

u10=u9;
u9=u8;
u8=u7;
u7=u6;
u6=u5;
u5=u4;
u4=u3;
u3=u2;
u2=u1;
u1=u;

y =(u1+u2+u3+u4+u5+u6+u7+u8+u9+u10)/10.0;

== matlab function Butunlesik Seyir Sistemi/Hesaplamalar/filter3 ==
  data: u input double; y output double
function y = f(u)
%#eml

persistent u1 u2 u3 u4 u5 u6 u7 u8 u9 u10

if isempty(u1)
    u1 = double(0);
    u2 = double(0);
    u3 = double(0);
    u4 = double(0);
    u5 = double(0);
    u6 = double(0);
    u7 = double(0);
    u8 = double(0);
    u9 = double(0);
    u10 = double(0);
end

u10=u9;
u9=u8;
u8=u7;
u7=u6;
u6=u5;
u5=u4;
u4=u3;
u3=u2;
u2=u1;
u1=u;

y =(u1+u2+u3+u4+u5+u6+u7+u8+u9+u10)/10.0;

== matlab function Butunlesik Seyir Sistemi/Hesaplamalar/filter4 ==
  data: u input double; y output double
function y = f(u)
%#eml

persistent u1 u2 u3 u4 u5 u6 u7 u8 u9 u10

if isempty(u1)
    u1 = double(0);
    u2 = double(0);
    u3 = double(0);
    u4 = double(0);
    u5 = double(0);
    u6 = double(0);
    u7 = double(0);
    u8 = double(0);
    u9 = double(0);
    u10 = double(0);
end

u10=u9;
u9=u8;
u8=u7;
u7=u6;
u6=u5;
u5=u4;
u4=u3;
u3=u2;
u2=u1;
u1=u;

y =(u1+u2+u3+u4+u5+u6+u7+u8+u9+u10)/10.0;

== matlab function Butunlesik Seyir Sistemi/Hesaplamalar/filter5 ==
  data: u input double; y output double
function y = f(u)
%#eml

persistent u1 u2 u3 u4 u5 u6 u7 u8 u9 u10 u11 u12 u13 u14 u15 u16 u17 u18 u19 u20

if isempty(u1)
    u1 = double(0);
    u2 = double(0);
    u3 = double(0);
    u4 = double(0);
    u5 = double(0);
    u6 = double(0);
    u7 = double(0);
    u8 = double(0);
    u9 = double(0);
    u10 = double(0);
    u11 = double(0);
    u12 = double(0);
    u13 = double(0);
    u14 = double(0);
    u15 = double(0);
    u16 = double(0);
    u17 = double(0);
    u18 = double(0);
    u19 = double(0);
    u20 = double(0);
end

u20=u19;
u19=u18;
u18=u17;
u17=u16;
u16=u15;
u15=u14;
u14=u13;
u13=u12;
u12=u11;
u11=u10;
u10=u9;
u9=u8;
u8=u7;
u7=u6;
u6=u5;
u5=u4;
u4=u3;
u3=u2;
u2=u1;
u1=u;

y =(u1+u2+u3+u4+u5+u6+u7+u8+u9+u10+u11+u12+u13+u14+u15+u16+u17+u18+u19+u20)/20.0;
